simulink model "sm_abbIrb120_1_RawImport"  (R2023a)
settings: Solver=VariableStepAuto  StartTime=0.0  StopTime=10.0  RelTol=1e-3
libraries: sm_lib x3, nesl_utility x1, fl_lib x1
settings Model: Creator=jjha  LastModifiedBy=abirdas
settings SimscapeCC: SimscapeLogType=all  SimscapeLogSimulationStatistics=on

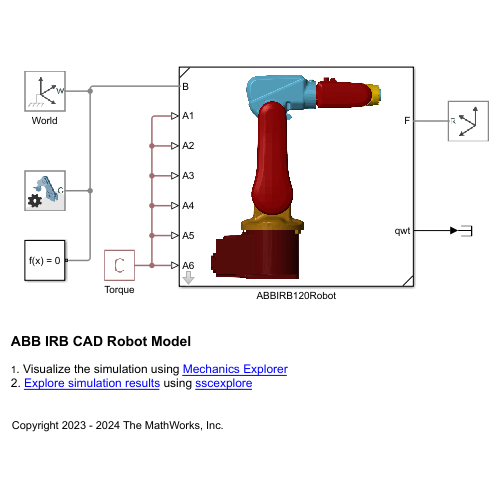
[thumbnail: Simulink's stored preview of the top-level diagram]
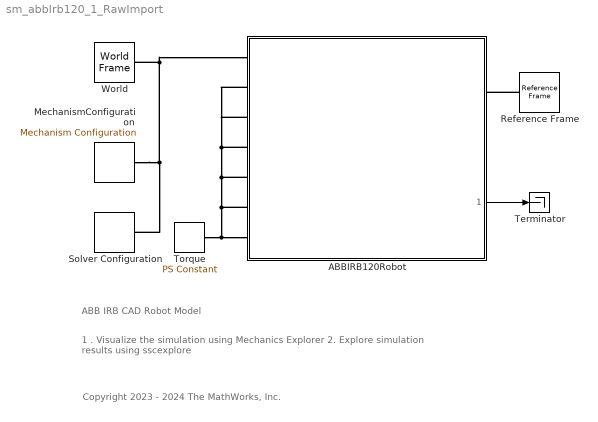
== system sm_abbIrb120_1_RawImport ==
  note: ABB IRB CAD Robot Model
  note: 1 . Visualize the simulation using Mechanics Explorer
      | 2. Explore simulation results using sscexplore
  note: Copyright 2023 - 2024 The MathWorks, Inc.
  ABBIRB120Robot : Subsystem  ReferencedSubsystem=ABBIRB120Robot  workflow=ones(1,6)
      settings: PortSchema="{\"entries\":[{\"content\":{\"sides\":[{\"content\":{\"connectorIds\":[\"LConn1\",\"LConn2\",\"LConn3\",\"LConn4\",\"LConn5\",\"LConn6\",\"LConn7\"]},\"type\":\"ConnectorPlacement.EquallySpacedRectSide\",\"uuid\":\"49a8ce80-385c-4ccb-9f7e-d5aab5db553d\"},{\"content\":{\"connectorIds\":[\"RConn1\",\"Out1\"],\"side\":\"RIGHT\"},\"type\":\"ConnectorPlacement.EquallySpacedRectSide\",\"uuid\":\"dfbdfbfc-5bd4-44cb-8e39-1f5ed0ef0e17\"},{\"content\":{\"side\":\"TOP\"},\"type\":\"ConnectorPlacement.EquallySpacedRectSide\",\"uuid\":\"57c1365f-1663-4513-9cc0-a14096685c3f\"}]},\"type\":\"ConnectorPlacement.EquallySpacedConnector\",\"uuid\":\"093e3139-792c-439d-b38f-5e7c8b0acc2e\"}],\"packageUris\":[\"http://schema.mathworks.com/mf0/Connector/R2020b\"],\"version\":\"1.0\"}"
  MechanismConfiguration : sm_lib/Utilities/Mechanism Configuration  UniformGravity=Constant  GravityVector=[0 0 -9.80665]  GravityVectorUnits=m/s^2  LinearizationDelta=0.001  JointModeTransitionNonlinearIterations=2
  Reference Frame : sm_lib/Frames and Transforms/Reference Frame
  Solver Configuration : nesl_utility/Solver Configuration  PhysicalDomain=network_engine_domain  SubClassName=solver  LeftPortType=input  RightPortType=generic  Tones=[]  Harmonics=[]  SimulateNoise=off  Profile=off  UseLocalSampling=off  EnableSwitchedLinearOptims=on  FrequencyDomain=off  UseCCode=off  RelTol=0.001  AbsTol=0.001  MinStep=1e-09  ToWorkspace=off  RevertToSquareIcSolve=off  NumHomotopyIterations=100  PhasorMode=off  PhasorModeNumHarmonics=1  ConsistencySolver=NEWTON_XTOL_AFTER_FTOL  IndexReductionMethod=DerivativeReplacement  DoDC=off  ResidualTolerance=1e-09  ConsistencyTolSource=GLOBAL  ConsistencyAbsTol=0.001  ConsistencyRelTol=0.001  ConsistencyTolFactor=0.001  UseLocalSolver=off  LocalSolverChoice=NE_BACKWARD_EULER_ADVANCER  ResolveIndetEquations=on  FunctionEvalNumThread=1  LocalSolverSampleTime=0.001  DoFixedCost=off  MaxNonlinIter=3  MaxModeIter=2  ComputeImpulses=off  ImpulseIterations=2  LinearAlgebra=auto  LinearAlgebraNumThread=0  EquationFormulation=NE_TIME_EF  DelaysMemoryBudget=1024  AutomaticFiltering=on  FilteringTimeConstant=0.001  PartitionStorageMethod=AS_NEEDED  PartitionMemoryBudget=1024  PartitionMethod=ROBUST
  Terminator : Terminator
  Torque : fl_lib/Physical Signals/Sources/PS Constant  constant=0 N*m
  World : sm_lib/Frames and Transforms/World Frame
  wires:
  ABBIRB120Robot/1 -> Terminator/1
  connections:
  MechanismConfiguration/RConn1 -- World/RConn1 -- ABBIRB120Robot/LConn1 -- Solver Configuration/RConn1
  Reference Frame/RConn1 -- ABBIRB120Robot/RConn1
  Torque/RConn1 -- ABBIRB120Robot/LConn2 -- ABBIRB120Robot/LConn3 -- ABBIRB120Robot/LConn4 -- ABBIRB120Robot/LConn5 -- ABBIRB120Robot/LConn6 -- ABBIRB120Robot/LConn7
